simulink library "DSX_Lib"  (R2020b)
settings: Solver=VariableStepAuto  StartTime=0.0  StopTime=10.0  RelTol=1e-3
undefined symbols (not defined in the file or in its folder): LF, serial
libraries: instrumentlib x5, simulink x1
settings Model: Creator=16047  LastModifiedBy=16047

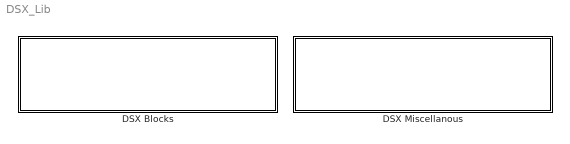
== system DSX_Lib ==
  DSX Blocks : Subsystem
      mask Display: image('team_logo_hires.jpg'); % Use "Edit Image" on toolstrip to change.
  DSX Miscellanous : Subsystem
      mask Display:
      | fprintf('Miscellaneous');
      | image('DAQ SIMPLE TEAM LOGO_whitebg.png',[0.01,0.65,0.3,0.3]);

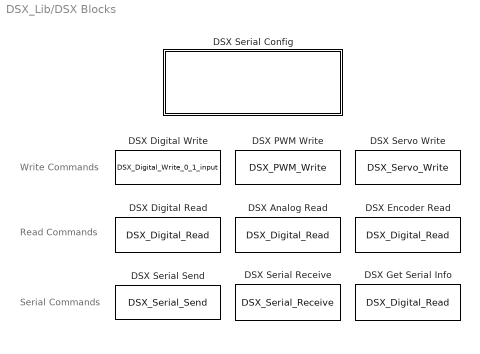
== system DSX_Lib/DSX Blocks ==
  note: Write Commands
  note: Read Commands
  note: Serial Commands
  DSX Analog Read : M-S-Function  FunctionName=DSX_Digital_Read  Parameters=double(receive_func),receive_loc  mask{receive_func=GPIO, receive_loc=2}
      mask prompts: receive_func "Function:"; receive_loc "Location:"
      mask init:
      | p = Simulink.Mask.get(gcb);
      | 
      | func = p.Parameters(1);
      | loc = p.Parameters(2);
      | 
      | assignin('base','loc_mask_init',loc.Value)
      | assignin('base','func_mask_init',func.Value)
      mask TypeOptions receive_func: GPIO | Encoder
      mask TypeOptions receive_loc: 2 | 4 | 7 | 10
      mask Display:
      | color('darkblue'); text(0.35, 0.5, 'DSX ', 'horizontalalignment', 'right');color('black'); text(0.35, 0.5, 'Analog Read', 'horizontalAlignment','left');
      | image('team_logo_lowerres.jpg',[0.65,0.75,1,1]);
  DSX Digital Read : M-S-Function  FunctionName=DSX_Digital_Read  Parameters=receive_loc  mask{receive_func=GPIO, receive_loc=2}
      mask prompts: receive_func "Function:"; receive_loc "Location:"
      mask init:
      | p = Simulink.Mask.get(gcb);
      | 
      | func = p.Parameters(1);
      | loc = p.Parameters(2);
      | 
      | assignin('base','loc_mask_init',loc.Value)
      | assignin('base','func_mask_init',func.Value)
      mask TypeOptions receive_func: GPIO | Encoder
      mask TypeOptions receive_loc: 2 | 4 | 7 | 10
      mask Display:
      | color('darkblue'); text(0.35, 0.5, 'DSX ', 'horizontalalignment', 'right');color('black'); text(0.35, 0.5, 'Digital Read', 'horizontalAlignment','left');
      | image('team_logo_lowerres.jpg',[0.65,0.75,1,1]);
  DSX Digital Write : M-S-Function  FunctionName=DSX_Digital_Write_0_1_input  Parameters=gpio_pin  mask{dtype=GPIO, gpio_pin=8, pwm_pin=8, pwm_freq=30}
      mask prompts: dtype "Digital Type:"; gpio_pin "Pin Number:"; pwm_pin "Pin Number :"; pwm_freq "Frequency : (Hz)"
      mask init:
      | % pwmbox=get_param(gcb,'enable_pwm');
      mask TypeOptions dtype: GPIO | PWM
      mask TypeOptions gpio_pin: 8 | 9 | 12 | 13
      mask TypeOptions pwm_pin: 8 | 9 | 12 | 13
      mask TypeOptions pwm_freq: 30 | 122 | 245 | 490 | 980 | 4000 | 32000
      mask DialogControl DescTextVar Prompt: Perform digital actions on your DSX.
      mask DialogControl Tab1 Prompt: High / Low
      mask DialogControl Tab2 Prompt: PWM
      mask Display:
      | color('darkblue'); text(0.40, 0.5, 'DSX ', 'horizontalalignment', 'right');color('black'); text(0.4, 0.5, 'Digital Write', 'horizontalAlignment','left');
      | image('team_logo_lowerres.jpg',[0.65,0.75,1,1]);
  DSX Encoder Read : M-S-Function  FunctionName=DSX_Digital_Read  Parameters=double(receive_func),receive_loc  mask{receive_func=GPIO, receive_loc=2}
      mask prompts: receive_func "Function:"; receive_loc "Location:"
      mask init:
      | p = Simulink.Mask.get(gcb);
      | 
      | func = p.Parameters(1);
      | loc = p.Parameters(2);
      | 
      | assignin('base','loc_mask_init',loc.Value)
      | assignin('base','func_mask_init',func.Value)
      mask TypeOptions receive_func: GPIO | Encoder
      mask TypeOptions receive_loc: 2 | 4 | 7 | 10
      mask Display:
      | color('darkblue'); text(0.35, 0.5, 'DSX ', 'horizontalalignment', 'right');color('black'); text(0.35, 0.5, 'Encoder Read', 'horizontalAlignment','left');
      | image('team_logo_lowerres.jpg',[0.65,0.75,1,1]);
  DSX Get Serial Info : M-S-Function  FunctionName=DSX_Digital_Read  Parameters=double(receive_func),receive_loc  mask{receive_func=GPIO, receive_loc=2}
      mask prompts: receive_func "Function:"; receive_loc "Location:"
      mask init:
      | p = Simulink.Mask.get(gcb);
      | 
      | func = p.Parameters(1);
      | loc = p.Parameters(2);
      | 
      | assignin('base','loc_mask_init',loc.Value)
      | assignin('base','func_mask_init',func.Value)
      mask TypeOptions receive_func: GPIO | Encoder
      mask TypeOptions receive_loc: 2 | 4 | 7 | 10
      mask Display:
      | color('darkblue'); text(0.4, 0.5, 'DSX ', 'horizontalalignment', 'right');color('black'); text(0.4, 0.5, 'Serial Info', 'horizontalAlignment','left');
      | image('team_logo_lowerres.jpg',[0.65,0.75,1,1]);
  DSX PWM Write : M-S-Function  FunctionName=DSX_PWM_Write  Parameters=pwm_pin,pwm_freq  mask{pwm_pin=3, pwm_freq=30}
      mask prompts: pwm_pin "Pin Number :"; pwm_freq "Frequency : (Hz)"
      mask init:
      | % pwmbox=get_param(gcb,'enable_pwm');
      mask TypeOptions pwm_pin: 3 | 5
      mask TypeOptions pwm_freq: 30 | 122 | 245 | 490 | 980 | 4000 | 32000
      mask DialogControl DescTextVar Prompt: Perform digital actions on your DSX.
      mask DialogControl Tab2 Prompt: PWM
      mask Display:
      | color('darkblue'); text(0.4, 0.5, 'DSX ', 'horizontalalignment', 'right');color('black'); text(0.4, 0.5, 'PWM Write', 'horizontalAlignment','left');
      | image('team_logo_lowerres.jpg',[0.65,0.75,1,1]);
  DSX Serial Config : Subsystem  mask{ComPort=COM1, BaudRate=9600}
      mask prompts: ComPort "Communication Port:"; BaudRate "Baud Rate:"
      mask init:
      | Serial_Config_callback('init');
      | 
      | p = Simulink.Mask.get(gcb);
      | 
      | com = p.Parameters(1);
      | 
      | baud = p.Parameters(2);
      | 
      | gcom = evalin('base','globalCom')
      | gbaud = num2str(evalin('base','globalBaud'))
      | [ports,numports]=Serial_Get_Ports();
      | 
      | % update com port menu with all available com ports
      | 
      | com.set('TypeOptions',ports); 
      | 
      | % update com port and baud rate
      | 
      | if strcmp(com.Value,gcom)
      |     Serial_Config_callback('update',com.Value,baud.Value);
      | end
      | if strcmp(baud.Value,gbaud)
      |     Serial_Config_callback('update',com.Value,baud.Value);
      | end
      mask TypeOptions ComPort: COM1 | COM5
      mask Callback ComPort:
      | % p = Simulink.Mask.get(gcb);
      | % com = p.Parameters(1);
      | % baud = p.Parameters(2);
      | % Serial_Config_callback('update',com.Value,baud.Value);
      mask TypeOptions BaudRate: 1200 | 2400 | 4800 | 9600 | 14400 | 19200 | 38400 | 57600 | 115200 | 128000 | 256000
      mask Callback BaudRate:
      | % p = Simulink.Mask.get(gcb);
      | % com = p.Parameters(1);
      | % baud = p.Parameters(2);
      | % Serial_Config_callback('update',com.Value,baud.Value);
      mask DialogControl DescGroupVar Prompt: DSX Serial Configure
      mask DialogControl DescTextVar Prompt: Configure your COM port specifications below.
      mask Display:
      | color('darkblue'); text(0.5, 0.85, 'DSX', 'horizontalalignment', 'center');color('black'); text(0.50, 0.15, 'Serial Configuration', 'horizontalAlignment','center');
      | image('team_logo_lowerres.jpg','center');
      | 
      | p = Simulink.Mask.get(gcb);
      | com = p.Parameters(1);
      | baud = p.Parameters(2);
      | 
      | %display things
      | try     %attempt to run code
      |     text(0.03,0.1,com.Value);
      | catch   %if an error occurs, address it and run this code
      |     com.set('Value','whack')
      |     text(0.03,0.1,com.Value)
      | end
      | 
      | try     %attempt to run code
      | 
      |     text(0.8,0.1,baud.Value);
      | catch   %if an error occurs, address it and run this code
      |     baud.set('Value','9600')
      |     text(0.03,0.1,baud.Value)
      | end
  DSX Serial Receive : M-S-Function  FunctionName=DSX_Serial_Receive  Parameters=double(receive_func),receive_loc  mask{receive_func=GPIO, receive_loc=2}
      mask prompts: receive_func "Function:"; receive_loc "Location:"
      mask init:
      | p = Simulink.Mask.get(gcb);
      | 
      | func = p.Parameters(1);
      | loc = p.Parameters(2);
      | 
      | assignin('base','loc_mask_init',loc.Value)
      | assignin('base','func_mask_init',func.Value)
      mask TypeOptions receive_func: GPIO | Encoder
      mask TypeOptions receive_loc: 2 | 4 | 7 | 10
      mask Display:
      | color('darkblue'); text(0.35, 0.5, 'DSX ', 'horizontalalignment', 'right');color('black'); text(0.35, 0.5, 'Serial Receive', 'horizontalAlignment','left');
      | image('team_logo_lowerres.jpg',[0.65,0.75,1,1]);
  DSX Serial Send : M-S-Function  FunctionName=DSX_Serial_Send  Parameters=1013100009
      mask Display:
      | color('darkblue'); text(0.40, 0.5, 'DSX ', 'horizontalalignment', 'right');color('black'); text(0.4, 0.5, 'Serial Send', 'horizontalAlignment','left');
      | image('team_logo_lowerres.jpg',[0.65,0.75,1,1]);
  DSX Servo Write : M-S-Function  FunctionName=DSX_Servo_Write  Parameters=servo_pin  mask{servo_pin=6}
      mask prompts: servo_pin "Pin Number:"
      mask init:
      | % pwmbox=get_param(gcb,'enable_pwm');
      mask TypeOptions servo_pin: 6
      mask DialogControl DescTextVar Prompt: Perform digital actions on your DSX.
      mask DialogControl Tab1 Prompt: Servo
      mask Display:
      | color('darkblue'); text(0.38, 0.5, 'DSX ', 'horizontalalignment', 'right');color('black'); text(0.38, 0.5, 'Servo Write', 'horizontalAlignment','left');
      | image('team_logo_lowerres.jpg',[0.65,0.75,1,1]);

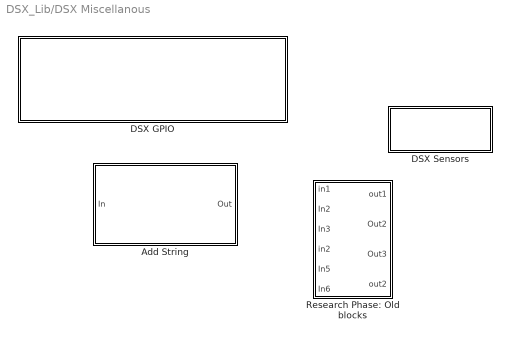
== system DSX_Lib/DSX Miscellanous ==
  Add String : Subsystem  mask(Add Delimiter){stringadd1=",", stringadd_index='After'}
      mask prompts: stringadd1 "String:"; stringadd_index "Where to add text:"
      mask TypeOptions stringadd1: String Constant/String
      mask TypeOptions stringadd_index: 'Before' | 'After'
      mask DialogControl DescTextVar Prompt: Insert your text before or after an input string.
      mask Display:
      | image('DAQ SIMPLE TEAM LOGO_whitebg.png',[0.01,0.7,0.6,0.5]); % Use "Edit Image" on toolstrip to change.
      | fprintf('Add String');
  DSX GPIO : Subsystem  StartFcn=|
      | if (contains(ComPortMenu,('COM')))
      |     ComPort = ComPortMenu; 
      | end
      mask Display: image('DAQ SIMPLE TEAM LOGO_whitebg.png'); % Use "Edit Image" on toolstrip to change.
  DSX Sensors : Subsystem
  Research Phase: Old blocks : Subsystem

== system DSX_Lib/DSX Blocks/DSX Serial Config ==

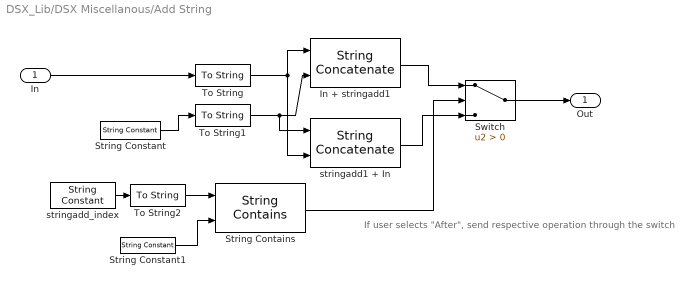
== system DSX_Lib/DSX Miscellanous/Add String ==
  note: If user selects "After", send respective operation through the switch
  In : Inport
  In + stringadd1 : StringConcatenate
  String Constant : StringConstant  String=stringadd1
  String Constant1 : StringConstant  String="\"After\""
  String Contains : StringContains
  Switch : Switch  Criteria=u2 > Threshold
  To String : ToString
  To String1 : ToString
  To String2 : ToString
  stringadd1 + In : StringConcatenate
  stringadd_index : StringConstant  String=stringadd_index
  Out : Outport
  wires:
  In/1 -> To String/1
  To String/1 -> stringadd1 + In/2, In + stringadd1/1
  String Constant/1 -> To String1/1
  To String1/1 -> In + stringadd1/2, stringadd1 + In/1
  String Constant1/1 -> String Contains/2
  In + stringadd1/1 -> Switch/1
  stringadd1 + In/1 -> Switch/3
  String Contains/1 -> Switch/2
  Switch/1 -> Out/1
  stringadd_index/1 -> To String2/1
  To String2/1 -> String Contains/1

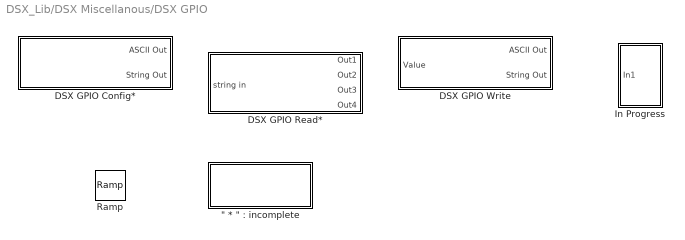
== system DSX_Lib/DSX Miscellanous/DSX GPIO ==
  "\" * \" : incomplete" : Subsystem
  DSX GPIO Config* : Subsystem  mask(DSX_GPIO_Write){a_pingroup=GPIOB, a_toggle_pingroup=off, gpio_type=digitalOut, a_pin=2}
      mask prompts: a_pingroup "Pin Group:"; a_toggle_pingroup "Toggle Sending"GPIOx""; gpio_type "GPIO Type:"; a_pin "Pin:"
      mask help: A general purpose GPIO block designed to communicate via serial with any MCU accepting DSX format commands.
      mask init:
      | set_param(gcb, 'MaskSelfModifiable', 'on');
      mask Help: web(https://youtu.be/dQw4w9WgXcQ)
      mask TypeOptions a_pingroup: GPIOA | GPIOB | GPIOC | GPIOD | GPIOE
      mask TypeOptions gpio_type: digitalIn | digitalOut | analogIn | analogOut
      mask TypeOptions a_pin: 1 | 2 | 3 | 4 | 5 | 6 | 7 | 8 | 9 | 10 | 11 | 12 | 13 | 14
      mask DialogControl DescGroupVar Prompt: DAQSimple
      mask DialogControl DescTextVar Prompt: Configure the GPIO pin of your choice:
      mask DialogControl Container5 Prompt: Manufacturer's Information
      mask DialogControl Control6 Prompt: This block was designed for the DSX by DAQSimple using Simulink.
      mask DialogControl Control6 Tooltip: whats up
      mask DialogControl Control7 Prompt: Author: Tim Saxon
      mask DialogControl Container3 Prompt: Format for Values:
      mask DialogControl Control3 Prompt: dio: 0 - 1
      mask DialogControl Control2 Prompt: pwm: 0-255
      mask DialogControl Control4 Prompt: servo: 0-180
      mask Display:
      | image('$imagefile',[0.1,0.1,0.8,0.8]);
      | text(0.4,0.1,'GPIO Config');
  DSX GPIO Read* : Subsystem  mask(DSX_GPIO_Write){a_pingroup=GPIOB, a_toggle_pingroup=off, a_function=digitalRead, pinNum=2}
      mask prompts: a_pingroup "Pin Group:"; a_toggle_pingroup "Toggle Sending"GPIOx""; a_function "Function:"; pinNum "Pin:"
      mask help: A general purpose GPIO block designed to communicate via serial with any MCU accepting DSX format commands.
      mask init:
      | set_param(gcb, 'MaskSelfModifiable', 'on');
      mask Help: web(https://youtu.be/dQw4w9WgXcQ)
      mask TypeOptions a_pingroup: GPIOA | GPIOB | GPIOC | GPIOD | GPIOE
      mask TypeOptions a_function: digitalRead | analogRead | getDioMode | encoderSpeed | encoderDir
      mask TypeOptions pinNum: 1 | 2 | 3 | 4 | 5 | 6 | 7 | 8 | 9 | 10 | 11 | 12 | 13 | 14
      mask DialogControl DescGroupVar Prompt: DAQSimple
      mask DialogControl DescTextVar Prompt: Configure your GPIO Read preferences:
      mask DialogControl Container5 Prompt: Manufacturer's Information
      mask DialogControl Control6 Prompt: This block was designed for the DSX by DAQSimple using Simulink.
      mask DialogControl Control6 Tooltip: whats up
      mask DialogControl Control7 Prompt: Author: Tim Saxon
      mask Display:
      | image('$imagefile',[0.1,0.1,0.8,0.8]);
      | text(0.4,0.1,'GPIO Read');
  DSX GPIO Write : Subsystem  StartFcn=|  StopFcn=|  mask(DSX_GPIO_Write){ComPortMenu=<Please select a port...>, ComPort=<Please select a port...>, EnableBlockingMode=on, Header=, Terminator=LF ('\n'), a_pingroup=GPIOB, a_toggle_pingroup=off, a_function=digitalWrite, a_pin=2}
      | % if (contains(ComPortMenu,('COM')))
      | %     ComPort = ComPortMenu; 
      | % end
      | % if (contains(ComPortMenu,('COM')))
      | %     ComPort = ComPortMenu; 
      | % end
      mask prompts: ComPortMenu "Communication port:"; ComPort "DummyPort:"; EnableBlockingMode "Enable blocking mode"; a_pingroup "Pin Group:"; a_toggle_pingroup "Send "GPIOx""; a_function "Function:"; a_pin "Pin:"
      mask help: A general purpose GPIO block designed to communicate via serial with any MCU accepting DSX format commands.
      mask init:
      | %set_param(gcb, 'MaskSelfModifiable', 'on');
      settings: PauseFcn=|
      | % if (contains(ComPortMenu,('COM')))
      | %     ComPort = ComPortMenu;
      | % end
      settings: ContinueFcn=|
      | % if (contains(ComPortMenu,('COM')))
      | %     ComPort = ComPortMenu;
      | % end
      mask Help: web(https://youtu.be/dQw4w9WgXcQ)
      mask TypeOptions ComPortMenu: Serial Send/ComPortMenu
      mask TypeOptions ComPort: Serial Send/ComPort | Serial Send/ObjConstructor
      mask TypeOptions EnableBlockingMode: Serial Send/EnableBlockingMode
      mask TypeOptions Header: Serial Send/Header
      mask TypeOptions Terminator: Serial Send/Terminator
      mask TypeOptions a_pingroup: GPIOA | GPIOB | GPIOC | GPIOD | GPIOE
      mask TypeOptions a_function: digitalWrite | pwm | pwm16 | servo
      mask TypeOptions a_pin: 1 | 2 | 3 | 4 | 5 | 6 | 7 | 8 | 9 | 10 | 11 | 12 | 13 | 14
      mask DialogControl DescGroupVar Prompt: DAQSimple
      mask DialogControl Control6 Prompt: Use this block to generate string commands for DSX GPIO serial communications.
      mask DialogControl Control6 Tooltip: whats up
      mask DialogControl Container6 Prompt: Advanced Settings
      mask DialogControl Container3 Prompt: Format for Values:
      mask DialogControl Control3 Prompt: dio: 0 - 1
      mask DialogControl Control2 Prompt: pwm: 0-255
      mask DialogControl Control4 Prompt: servo: 0-180
      mask DialogControl Container5 Prompt: Manufacturer's Information
      mask DialogControl Control12 Prompt: DAQSimple is a company founded by SFU students.
      mask DialogControl Control7 Prompt: Author: Tim Saxon
      mask Display:
      | image('$imagefile',[0.1,0.1,0.8,0.8]);
      | text(0.4,0.1,'GPIO Write');
  In Progress : Subsystem
  Ramp : simulink/Sources/Ramp  slope=1  start=0  InitialOutput=0

== system DSX_Lib/DSX Miscellanous/DSX Sensors ==

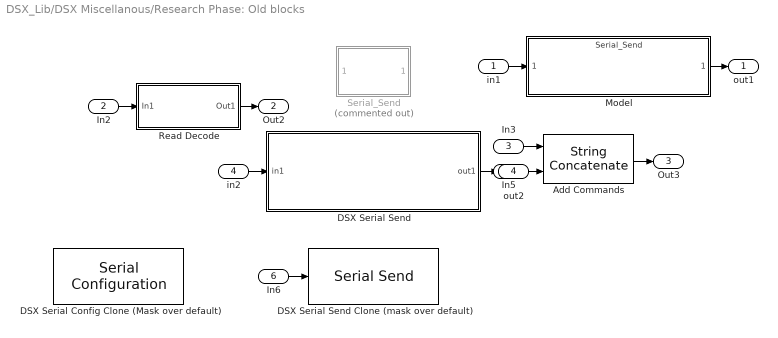
== system DSX_Lib/DSX Miscellanous/Research Phase: Old blocks ==
  in1 : Inport
  In2 : Inport  Port=2
  In3 : Inport  Port=3
  in2 : Inport  Port=4
  In5 : Inport  Port=5
  In6 : Inport  Port=6
  Add Commands : StringConcatenate  Inputs=Inputs  mask{Inputs=2, OutDataTypeStr=string}
      mask prompts: Inputs "Simulink:blkprm_prompts:ConcatNumInputs"; OutDataTypeStr "Simulink:blkprm_prompts:OUTPUT_UNIFIEDDATATYPE"
      mask TypeOptions Inputs: Inputs
      mask TypeOptions OutDataTypeStr: OutDataTypeStr
      mask DialogControl DescTextVar Prompt: Concatenate all inputs into a single output
      mask DialogControl Inputs Prompt: Number of inputs:
      mask DialogControl Container3 Prompt: Advanced settings
      mask DialogControl OutDataTypeStr Prompt: Output data type:
  DSX Serial Config Clone (Mask over default) : instrumentlib/Serial Configuration  Priority=-200000  ComPortMenu=<Please select a port...>  ComPort=<Please select a port...>  BaudRate=9600  DataBits=8  Parity=none  StopBits=1  FlowControl=none  Timeout=10  ByteOrder=LittleEndian
  DSX Serial Send : Subsystem
      mask init:
      | try
      | O = evalin('caller','O');
      | T = evalin('caller','T');
      | catch
      | end
      | try
      |     evalin('base','DSX')
      |     disp('test2')
      | catch
      |     Serial_Send_callback('init');
      |     disp('test2')
      | end
      | % p = Simulink.Mask.get(gcb);
      | % com = p.Parameters(1);
      | % baud = p.Parameters(2);
      | if exist('O')
      |     message = O;
      |     dispp('message: ');
      |     dispp(message);
      | else
      | message = 'dsx,digitalWrite,13,0\n';% StringIn
      | dispp('no input message, led off');
      | end
      | 
      | % com.set('TypeOptions',ports);
      | 
      | % Serial_Config_callback('update_com',com.Value);
      | % Serial_Config_callback('update_baud',baud.Value);
      | 
      | Serial_Send_callback('send',message);
      mask DialogControl Control2 Prompt: DSX.
  DSX Serial Send Clone (mask over default) : instrumentlib/Serial Send  ComPortMenu=<Please select a port...>  ComPort=<Please select a port...>  Terminator=<none>  EnableBlockingMode=off
  Model : ModelReference  ModelNameDialog=Serial_Send.slx  SimulationMode=Normal  ShowModelTerminatePort=on  ModelReferenceVersion=1.6
      mask init:
      | blocktobase();
      | try
      |     evalin('base','DSX')
      | catch
      |     Serial_Send_callback('init');
      | end
      | % p = Simulink.Mask.get(gcb);
      | % com = p.Parameters(1);
      | % baud = p.Parameters(2);
      | if exist('sendOut')
      |     message = sendOut;
      |     dispp('message: ');
      |     dispp(message);
      | else
      | message = 'dsx,digitalWrite,13,0\n';% StringIn
      | dispp('no input message, led off');
      | end
      | 
      | % com.set('TypeOptions',ports);
      | 
      | % Serial_Config_callback('update_com',com.Value);
      | % Serial_Config_callback('update_baud',baud.Value);
      | 
      | Serial_Send_callback('send',message);
      mask DialogControl Control2 Prompt: Serial Send model
  Read Decode : Subsystem
  Serial_Send : MATLAB Function  Commented=on  TreatAsAtomicUnit=on
  out1 : Outport
  Out2 : Outport  Port=2
  Out3 : Outport  Port=3
  out2 : Outport  Port=4
  wires:
  Read Decode/1(Out1) -> Out2/1
  In6/1 -> DSX Serial Send Clone (mask over default)/1
  in2/1 -> DSX Serial Send/1(in1)
  in1/1 -> Model/1
  Add Commands/1 -> Out3/1
  In2/1 -> Read Decode/1(In1)
  Model/1 -> out1/1
  DSX Serial Send/1(out1) -> out2/1
  In5/1 -> Add Commands/2
  In3/1 -> Add Commands/1

== system DSX_Lib/DSX Miscellanous/DSX GPIO/" * " : incomplete ==
  wires:
  ? -> ?

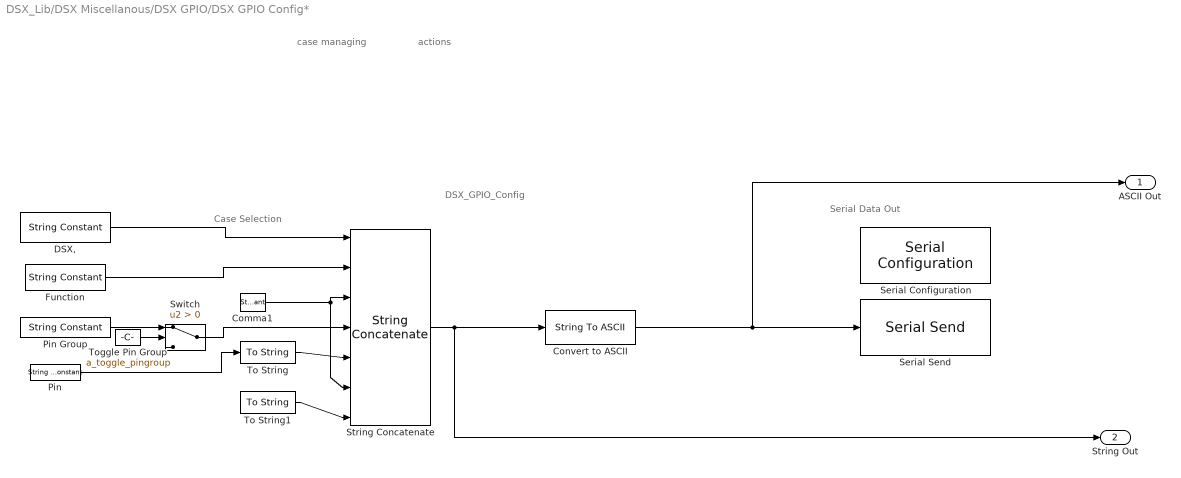
== system DSX_Lib/DSX Miscellanous/DSX GPIO/DSX GPIO Config* ==
  note: actions
  note: case managing
  note: DSX_GPIO_Config
  note: Case Selection
  note: Serial Data Out
  Comma1 : StringConstant  String="\",\""
  Convert to ASCII : StringToASCII
  DSX, : StringConstant  String="\"dsx,\""
  Function : StringConstant  String=gpio_type
  Pin : StringConstant  String=a_pin
  Pin Group : StringConstant  String=a_pingroup
  Serial Configuration : instrumentlib/Serial Configuration  Priority=-200000  ComPortMenu=<Please select a port...>  ComPort=COM5  ObjConstructor=serial('COM5');  BaudRate=74880  DataBits=8  Parity=none  StopBits=1  FlowControl=none  Timeout=10  ByteOrder=LittleEndian
  Serial Send : instrumentlib/Serial Send  ComPortMenu=<Please select a port...>  ComPort=COM5  ObjConstructor=serial('COM5');  Terminator=LF ('\n')  EnableBlockingMode=on
  String Concatenate : StringConcatenate  Inputs=7
  Switch : Switch  Criteria=u2 > Threshold
  To String : ToString
  To String1 : ToString
  Toggle Pin Group : Constant  Value=a_toggle_pingroup
  ASCII Out : Outport
  String Out : Outport  Port=2
  wires:
  String Concatenate/1 -> Convert to ASCII/1, String Out/1
  Convert to ASCII/1 -> ASCII Out/1, Serial Send/1
  Pin/1 -> To String/1
  DSX,/1 -> String Concatenate/1
  Function/1 -> String Concatenate/2
  To String/1 -> String Concatenate/5
  To String1/1 -> String Concatenate/7
  Comma1/1 -> String Concatenate/6, String Concatenate/3
  Pin Group/1 -> Switch/1
  Toggle Pin Group/1 -> Switch/2
  Switch/1 -> String Concatenate/4

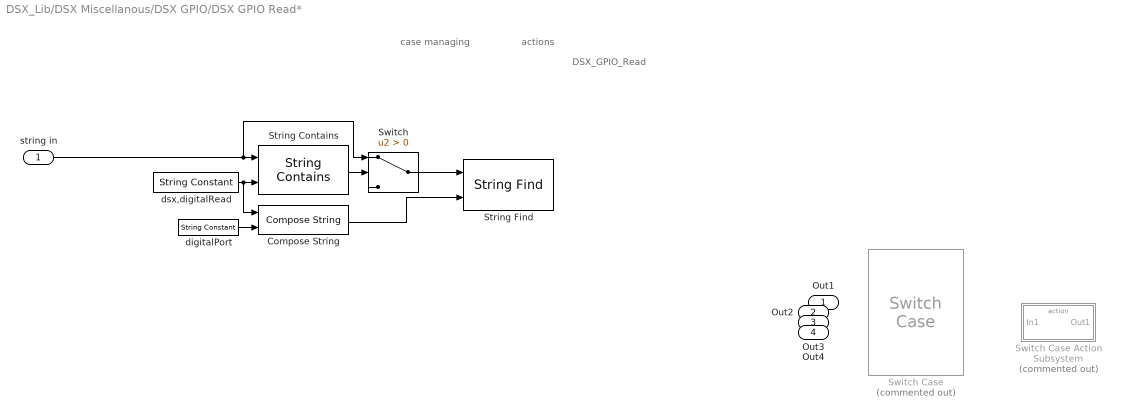
== system DSX_Lib/DSX Miscellanous/DSX GPIO/DSX GPIO Read* ==
  note: actions
  note: case managing
  note: DSX_GPIO_Read
  string in : Inport
  Compose String : ComposeString  Format="\"%s,%s\""
  String Contains : StringContains
  String Find : StringFind
  Switch : Switch  Criteria=u2 > Threshold
  Switch Case : SwitchCase  Commented=on  CaseConditions={1,2,3,4,5}
  Switch Case Action Subsystem : Subsystem  Commented=on  TreatAsAtomicUnit=on
  digitalPort : StringConstant  String=pinNum
  dsx,digitalRead : StringConstant  String="\"dsx,digitalRead\""
  Out1 : Outport
  Out2 : Outport  Port=2
  Out3 : Outport  Port=3
  Out4 : Outport  Port=4
  wires:
  ? -> Out1/1
  ? -> Out2/1
  ? -> Out3/1
  ? -> Out4/1
  string in/1 -> Switch/1, String Contains/1
  dsx,digitalRead/1 -> Compose String/1, String Contains/2
  String Contains/1 -> Switch/2
  Switch/1 -> String Find/1
  Compose String/1 -> String Find/2
  digitalPort/1 -> Compose String/2

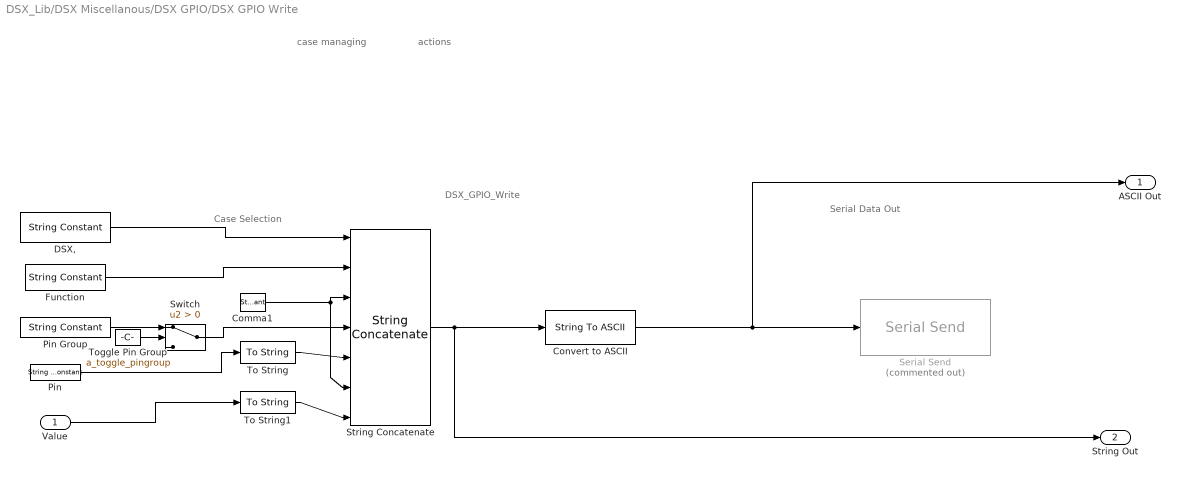
== system DSX_Lib/DSX Miscellanous/DSX GPIO/DSX GPIO Write ==
  note: actions
  note: case managing
  note: DSX_GPIO_Write
  note: Case Selection
  note: Serial Data Out
  Value : Inport
  Comma1 : StringConstant  String="\",\""
  Convert to ASCII : StringToASCII
  DSX, : StringConstant  String="\"dsx,\""
  Function : StringConstant  String=a_function
  Pin : StringConstant  String=a_pin
  Pin Group : StringConstant  String=a_pingroup
  Serial Send : instrumentlib/Serial Send  Commented=on  ComPortMenu=<Please select a port...>  ComPort=<Please select a port...>  ObjConstructor=<Please select a port...>  Terminator=LF ('\n')  EnableBlockingMode=on
  String Concatenate : StringConcatenate  Inputs=7
  Switch : Switch  Criteria=u2 > Threshold
  To String : ToString
  To String1 : ToString
  Toggle Pin Group : Constant  Value=a_toggle_pingroup
  ASCII Out : Outport
  String Out : Outport  Port=2
  wires:
  String Concatenate/1 -> Convert to ASCII/1, String Out/1
  Convert to ASCII/1 -> ASCII Out/1, Serial Send/1
  Pin/1 -> To String/1
  Value/1 -> To String1/1
  DSX,/1 -> String Concatenate/1
  Function/1 -> String Concatenate/2
  To String/1 -> String Concatenate/5
  To String1/1 -> String Concatenate/7
  Comma1/1 -> String Concatenate/6, String Concatenate/3
  Pin Group/1 -> Switch/1
  Toggle Pin Group/1 -> Switch/2
  Switch/1 -> String Concatenate/4

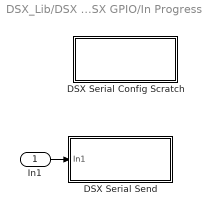
== system DSX_Lib/DSX Miscellanous/DSX GPIO/In Progress ==
  In1 : Inport
  DSX Serial Config Scratch : Subsystem  mask{DSXComPort=<Select a port...>, BaudRate=9600}
      mask prompts: DSXComPort "COM Port:"; BaudRate "Baud Rate:"
      mask init:
      | if(contains(DSXComPort,('COM')))
      |     s = serialport(DSXComPort,str2double(BaudRate))
      | end
      mask TypeOptions DSXComPort: <Select a port...> | COM1 | COM2 | COM3 | COM4 | COM5 | COM6 | COM7 | COM8 | COM9
      mask TypeOptions BaudRate: 1200 | 4800 | 9600 | 19200 | 38400 | 57600 | 115200
  DSX Serial Send : Subsystem
  wires:
  In1/1 -> DSX Serial Send/1(In1)

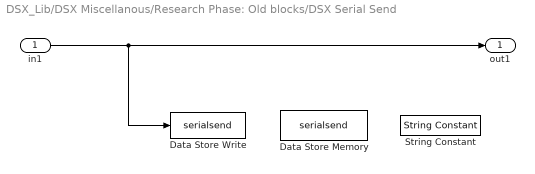
== system DSX_Lib/DSX Miscellanous/Research Phase: Old blocks/DSX Serial Send ==
  in1 : Inport
  Data Store Memory : DataStoreMemory  DataStoreName=serialsend  ReadBeforeWriteMsg=warning  WriteAfterWriteMsg=warning  WriteAfterReadMsg=warning  ShowAdditionalParam=off
  Data Store Write : DataStoreWrite  DataStoreName=serialsend  DataStoreElements=serialsend
  String Constant : StringConstant  String=serialsend
  out1 : Outport
  wires:
  in1/1 -> Data Store Write/1, out1/1

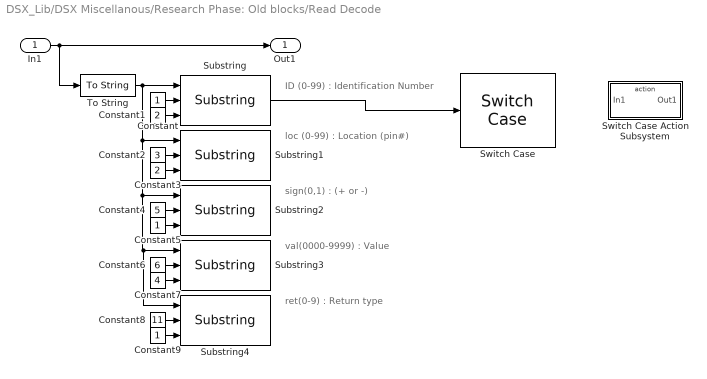
== system DSX_Lib/DSX Miscellanous/Research Phase: Old blocks/Read Decode ==
  note: ID (0-99) : Identification Number
  note: loc (0-99) : Location (pin#)
  note: sign(0,1) : (+ or -)
  note: val(0000-9999) : Value
  note: ret(0-9) : Return type
  In1 : Inport
  Constant : Constant
  Constant1 : Constant  Value=2
  Constant2 : Constant  Value=3
  Constant3 : Constant  Value=2
  Constant4 : Constant  Value=5
  Constant5 : Constant
  Constant6 : Constant  Value=6
  Constant7 : Constant  Value=4
  Constant8 : Constant  Value=11
  Constant9 : Constant
  Substring{,1..4} (5 alike) : Substring
  Switch Case : SwitchCase  CaseConditions={(00),(01),(02)}
  Switch Case Action Subsystem : Subsystem  TreatAsAtomicUnit=on
  To String : ToString
  Out1 : Outport
  wires:
  In1/1 -> To String/1, Out1/1
  To String/1 -> Substring4/1, Substring3/1, Substring2/1, Substring1/1, Substring/1
  Constant/1 -> Substring/2
  Constant1/1 -> Substring/3
  Constant3/1 -> Substring1/3
  Constant2/1 -> Substring1/2
  Constant4/1 -> Substring2/2
  Constant5/1 -> Substring2/3
  Constant7/1 -> Substring3/3
  Constant6/1 -> Substring3/2
  Constant8/1 -> Substring4/2
  Constant9/1 -> Substring4/3
  Substring/1 -> Switch Case/1

== system DSX_Lib/DSX Miscellanous/DSX GPIO/DSX GPIO Read*/Switch Case Action Subsystem ==
  In1 : Inport
  Action Port : ActionPort
  Out1 : Outport
  wires:
  In1/1 -> Out1/1

== system DSX_Lib/DSX Miscellanous/DSX GPIO/In Progress/DSX Serial Config Scratch ==

== system DSX_Lib/DSX Miscellanous/DSX GPIO/In Progress/DSX Serial Send ==
  In1 : Inport

== system DSX_Lib/DSX Miscellanous/Research Phase: Old blocks/Read Decode/Switch Case Action Subsystem ==
  In1 : Inport
  Action Port : ActionPort
  Out1 : Outport
  wires:
  In1/1 -> Out1/1

== matlab function DSX_Lib/DSX Miscellanous/Research Phase: Old blocks/Serial_Send ==
  data: stringIn input; stringOut output
function stringOut = fcn(stringIn)
eval(Serial_Send_callback('init'));

if ~isstring(stringIn)
    stringIn=string(stringIn);
end
eval(Serial_Send_callback('send',stringIn));
stringOut = stringIn;
end %function
